simulink model "Ctrl_For_HRV_alpha_reversal_harness"  (R2024b)
settings: Solver=ode4  StartTime=0.0  StopTime=100  FixedStep=0.02  RelTol=1e-3
InitFcn:
  | Parameter;
values from neighbouring files (symbols this model uses):
  h_alpha = 0.02    [Data_0.mat]    (also in Parameter.m)
  h_beta = 0.02    [Data_0.mat]    (also in Parameter.m)
  h_miu = 0.02    [Data_0.mat]    (also in Parameter.m)
  h_p = 0.02    [Data_0.mat]    (also in Parameter.m)
  h_q = 0.02    [Data_0.mat]    (also in Parameter.m)
  h_r = 0.02    [Data_0.mat]    (also in Parameter.m)
  r_alpha = 0.04    [Data_0.mat]    (also in Parameter.m)
  r_beta = 0.04    [Data_0.mat]    (also in Parameter.m)
  r_miu = 0.03    [Data_0.mat]    (also in Parameter.m = 0.24)
  r_p = 1.28    [Data_0.mat]    (also in Parameter.m)
  r_q = 1.28    [Data_0.mat]    (also in Parameter.m)
  r_r = 1.28    [Data_0.mat]    (also in Parameter.m)
  xishu = 0.3    [Data_0.mat]    (also in Parameter.m = 0)
  xishu_D_0 = 0.3    [Parameter.m]
  xishu_L_0 = 0.2    [Parameter.m]
  xishu_l_0 = 0.23    [Parameter.m]
  xishu_m_0 = 0.17    [Parameter.m]
  xishu_n_0 = 0.09    [Parameter.m]
  xishu_Y_0 = 0.14    [Parameter.m]
undefined symbols (not defined in the file or in its folder): AngleRate_Controller, fhan, FlowAngle_Controller
libraries: simulink x12
settings Model: Creator=BinRen  LastModifiedBy=DuY
settings SolverCC: AlgebraicLoopSolver=TrustRegion
settings DataIOCC: SaveFormat=StructureWithTime  SaveState=on  TimeSaveName=time
settings DebuggingCC: UnconnectedInputMsg=warning  UnconnectedOutputMsg=warning  UnconnectedLineMsg=warning
settings ModelReferenceCC: EnableRefExpFcnMdlSchedulingChecks=on
settings RTWCC: GPUComputeCapability=3.5  DLArmComputeVersion=19.05

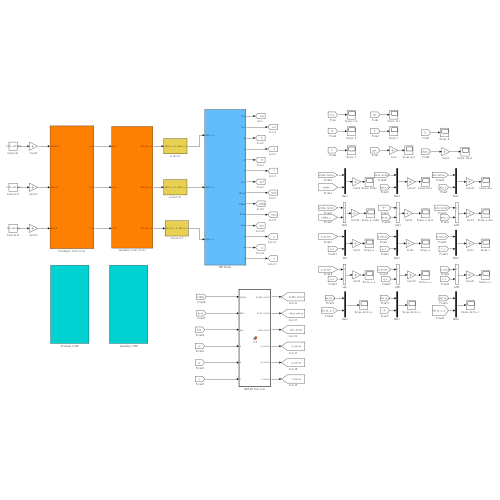
[thumbnail: Simulink's stored preview of the top-level diagram]
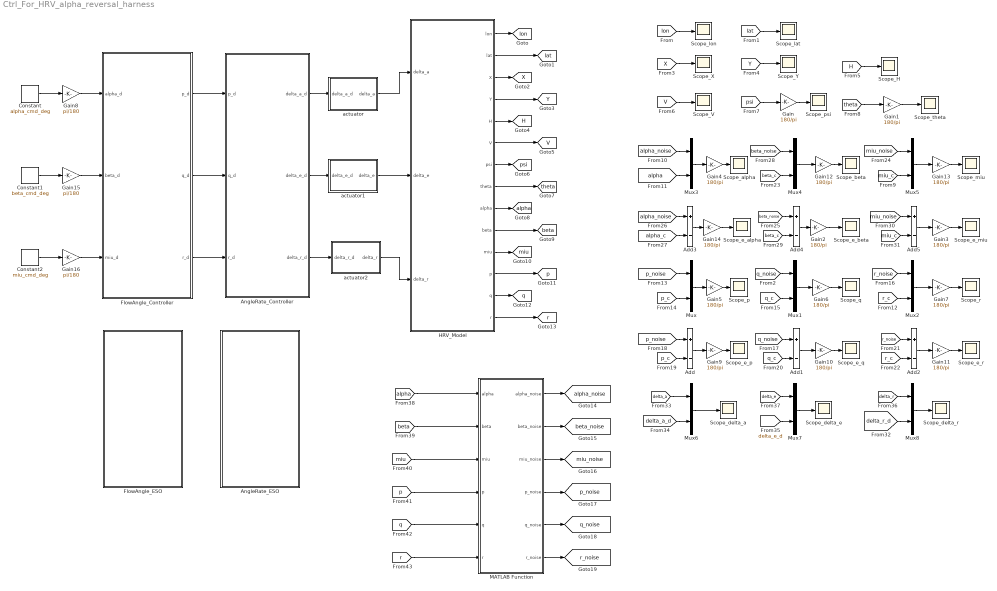
== system Ctrl_For_HRV_alpha_reversal_harness ==
  Add{,1..5} (6 alike) : Sum  Inputs=+-
  AngleRate_Controller : Subsystem
  AngleRate_ESO : Subsystem
  Constant : FromWorkspace  VariableName=alpha_cmd_deg
  Constant1 : FromWorkspace  VariableName=beta_cmd_deg
  Constant2 : FromWorkspace  VariableName=miu_cmd_deg
  FlowAngle_Controller : Subsystem
  FlowAngle_ESO : Subsystem
  Gain{,1..7,9..14} (14 alike) : Gain  Gain=180/pi
  Gain15 : Gain  Gain=pi/180
  Gain16 : Gain  Gain=pi/180
  Gain8 : Gain  Gain=pi/180
  HRV_Model : Subsystem
  MATLAB Function : MATLAB Function  TreatAsAtomicUnit=on
  Mux{,1..8} (9 alike) : Mux  Inputs=2
  Scope_H : Scope
  Scope_V : Scope
  Scope_X : Scope
  Scope_Y : Scope
  Scope_alpha : Scope
  Scope_beta : Scope
  Scope_delta_a : Scope
  Scope_delta_e : Scope
  Scope_delta_r : Scope
  Scope_e_alpha : Scope
  Scope_e_beta : Scope
  Scope_e_miu : Scope
  Scope_e_p : Scope
  Scope_e_q : Scope
  Scope_e_r : Scope
  Scope_lat : Scope
  Scope_lon : Scope
  Scope_miu : Scope
  Scope_p : Scope
  Scope_psi : Scope
  Scope_q : Scope
  Scope_r : Scope
  Scope_theta : Scope
  actuator : Subsystem
  actuator1 : Subsystem
  actuator2 : Subsystem
  tag scope: H=global, V=global, X=global, Y=global, alpha=global, alpha_noise=global, beta=global, beta_noise=global, lat=global, lon=global, miu=global, miu_noise=global, p=global, p_noise=global, psi=global, q=global, q_noise=global, r=global, r_noise=global, theta=global
  wires:
  HRV_Model/1(lon) -> [lon]
  HRV_Model/2(lat) -> [lat]
  HRV_Model/4(Y) -> [Y]
  HRV_Model/3(X) -> [X]
  HRV_Model/7(psi) -> [psi]
  HRV_Model/8(theta) -> [theta]
  HRV_Model/6(V) -> [V]
  HRV_Model/5(H) -> [H]
  HRV_Model/13(q) -> [q]
  HRV_Model/14(r) -> [r]
  HRV_Model/11(miu) -> [miu]
  HRV_Model/12(p) -> [p]
  HRV_Model/10(beta) -> [beta]
  HRV_Model/9(alpha) -> [alpha]
  [lon] -> Scope_lon/1
  [lat] -> Scope_lat/1
  [H] -> Scope_H/1
  [Y] -> Scope_Y/1
  [X] -> Scope_X/1
  [V] -> Scope_V/1
  [psi] -> Gain/1
  Gain/1 -> Scope_psi/1
  Gain1/1 -> Scope_theta/1
  [theta] -> Gain1/1
  Gain5/1 -> Scope_p/1
  Gain6/1 -> Scope_q/1
  Gain7/1 -> Scope_r/1
  actuator/1(delta_a) -> HRV_Model/1(delta_a)
  actuator1/1(delta_e) -> HRV_Model/2(delta_e)
  actuator2/1(delta_r) -> HRV_Model/3(delta_r)
  AngleRate_Controller/2(delta_e_d) -> actuator1/1(delta_e_d)
  [p_noise] -> Mux/1
  Mux/1 -> Gain5/1
  [p_c] -> Mux/2
  [q_c] -> Mux1/2
  [q_noise] -> Mux1/1
  Mux1/1 -> Gain6/1
  Mux2/1 -> Gain7/1
  [r_noise] -> Mux2/1
  [r_c] -> Mux2/2
  Gain11/1 -> Scope_e_r/1
  Gain10/1 -> Scope_e_q/1
  Gain9/1 -> Scope_e_p/1
  [p_c] -> Add/2
  [p_noise] -> Add/1
  Add/1 -> Gain9/1
  Add1/1 -> Gain10/1
  [q_noise] -> Add1/1
  [q_c] -> Add1/2
  [r_c] -> Add2/2
  [r_noise] -> Add2/1
  Add2/1 -> Gain11/1
  Add5/1 -> Gain3/1
  [miu_noise] -> Add5/1
  [miu_c] -> Add5/2
  [beta_c] -> Add4/2
  [beta_noise] -> Add4/1
  Add4/1 -> Gain2/1
  Add3/1 -> Gain14/1
  [alpha_noise] -> Add3/1
  [alpha_c] -> Add3/2
  Gain14/1 -> Scope_e_alpha/1
  Gain2/1 -> Scope_e_beta/1
  Gain3/1 -> Scope_e_miu/1
  [miu_c] -> Mux5/2
  [miu_noise] -> Mux5/1
  Mux5/1 -> Gain13/1
  Mux4/1 -> Gain12/1
  [beta_noise] -> Mux4/1
  [beta_c] -> Mux4/2
  [alpha] -> Mux3/2
  Mux3/1 -> Gain4/1
  [alpha_noise] -> Mux3/1
  Gain13/1 -> Scope_miu/1
  Gain12/1 -> Scope_beta/1
  Gain4/1 -> Scope_alpha/1
  Gain8/1 -> FlowAngle_Controller/1(alpha_d)
  [delta_r_d] -> Mux8/2
  [delta_r] -> Mux8/1
  [delta_e] -> Mux7/1
  [delta_e_d] -> Mux7/2
  [delta_a_d] -> Mux6/2
  [delta_a] -> Mux6/1
  Mux8/1 -> Scope_delta_r/1
  Mux7/1 -> Scope_delta_e/1
  Mux6/1 -> Scope_delta_a/1
  FlowAngle_Controller/1(p_d) -> AngleRate_Controller/1(p_d)
  FlowAngle_Controller/2(q_d) -> AngleRate_Controller/2(q_d)
  FlowAngle_Controller/3(r_d) -> AngleRate_Controller/3(r_d)
  Gain15/1 -> FlowAngle_Controller/2(beta_d)
  Gain16/1 -> FlowAngle_Controller/3(miu_d)
  AngleRate_Controller/3(delta_r_d) -> actuator2/1(delta_r_d)
  AngleRate_Controller/1(delta_a_d) -> actuator/1(delta_a_d)
  MATLAB Function/1(alpha_noise) -> [alpha_noise]
  [alpha] -> MATLAB Function/1(alpha)
  [beta] -> MATLAB Function/2(beta)
  [miu] -> MATLAB Function/3(miu)
  [p] -> MATLAB Function/4(p)
  [q] -> MATLAB Function/5(q)
  [r] -> MATLAB Function/6(r)
  MATLAB Function/2(beta_noise) -> [beta_noise]
  MATLAB Function/3(miu_noise) -> [miu_noise]
  MATLAB Function/4(p_noise) -> [p_noise]
  MATLAB Function/5(q_noise) -> [q_noise]
  MATLAB Function/6(r_noise) -> [r_noise]
  Constant/1 -> Gain8/1
  Constant1/1 -> Gain15/1
  Constant2/1 -> Gain16/1

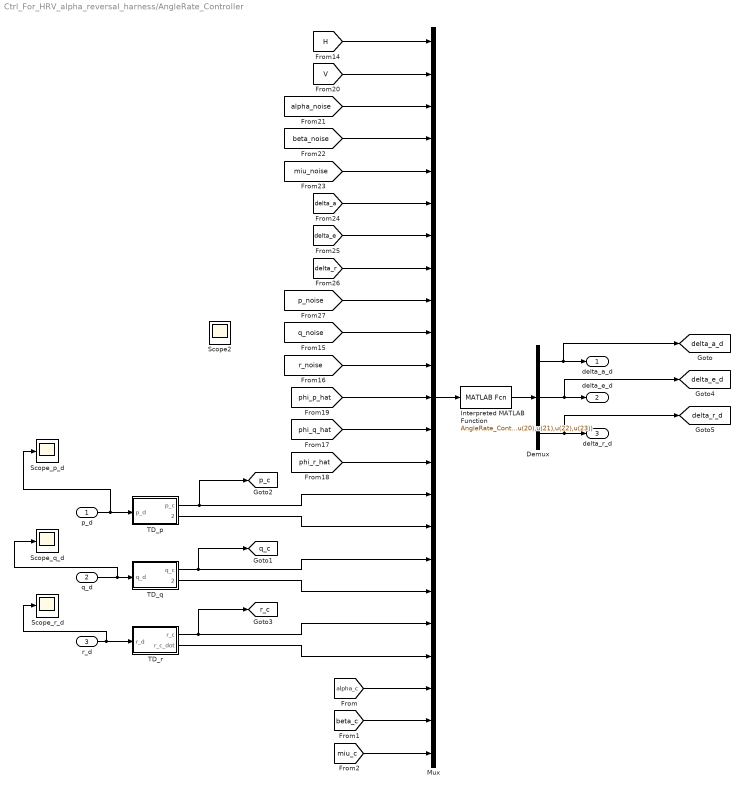
== system Ctrl_For_HRV_alpha_reversal_harness/AngleRate_Controller ==
  p_d : Inport
  q_d : Inport  Port=2
  r_d : Inport  Port=3
  Demux : Demux  Outputs=3
  Interpreted MATLAB Function : MATLABFcn  MATLABFcn=AngleRate_Controller(u(1),u(2),u(3),u(4),u(5),u(6),u(7),u(8),u(9),u(10),u(11),u(12),u(13),u(14),u(15),u(16),u(17),u(18),u(19),u(20),u(21),u(22),u(23))  OutputDimensions=3
  Mux : Mux  Inputs=23
  Scope2 : Scope
  Scope_p_d : Scope
  Scope_q_d : Scope
  Scope_r_d : Scope
  TD_p : Subsystem
  TD_q : Subsystem
  TD_r : Subsystem
  delta_a_d : Outport
  delta_e_d : Outport  Port=2
  delta_r_d : Outport  Port=3
  tag scope: delta_a_d=global, delta_e_d=global, delta_r_d=global, p_c=global, q_c=global, r_c=global
  wires:
  [miu_noise] -> Mux/5
  [beta_noise] -> Mux/4
  TD_r/1(r_c) -> [r_c], Mux/19
  TD_p/2(p_c_dot) -> Mux/16
  TD_q/2(q_c_dot) -> Mux/18
  [q_noise] -> Mux/10
  TD_q/1(q_c) -> [q_c], Mux/17
  TD_r/2(r_c_dot) -> Mux/20
  [r_noise] -> Mux/11
  [H] -> Mux/1
  [p_noise] -> Mux/9
  [V] -> Mux/2
  [alpha_noise] -> Mux/3
  Mux/1 -> Interpreted MATLAB Function/1
  Interpreted MATLAB Function/1 -> Demux/1
  [delta_a] -> Mux/6
  [delta_r] -> Mux/8
  [delta_e] -> Mux/7
  TD_p/1(p_c) -> [p_c], Mux/15
  Demux/3 -> [delta_r_d], delta_r_d/1
  r_d/1 -> Scope_r_d/1, TD_r/1(r_d)
  Demux/2 -> [delta_e_d], delta_e_d/1
  Demux/1 -> [delta_a_d], delta_a_d/1
  q_d/1 -> Scope_q_d/1, TD_q/1(q_d)
  p_d/1 -> Scope_p_d/1, TD_p/1(p_d)
  [phi_p_hat] -> Mux/12
  [phi_q_hat] -> Mux/13
  [phi_r_hat] -> Mux/14
  [alpha_c] -> Mux/21
  [beta_c] -> Mux/22
  [miu_c] -> Mux/23

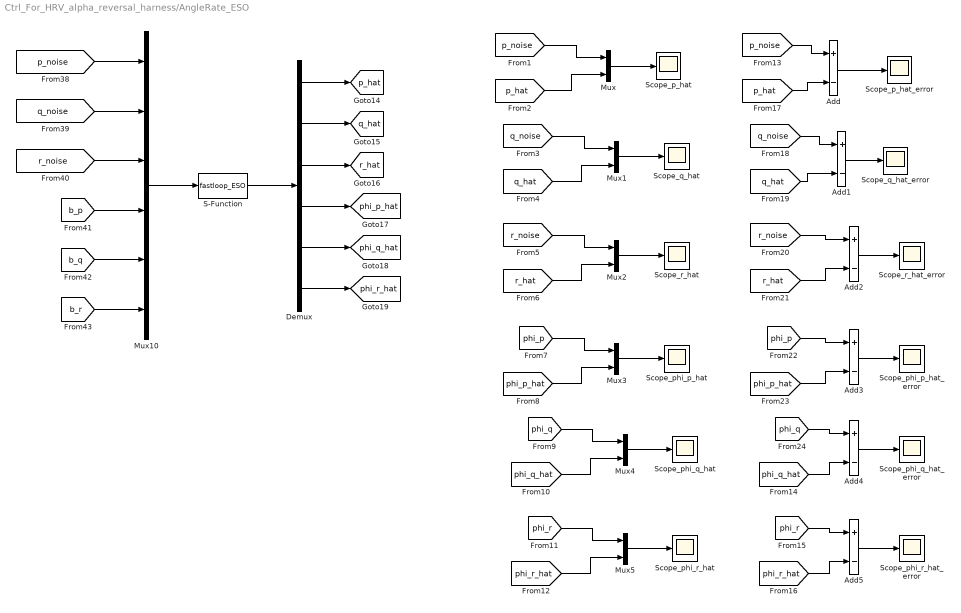
== system Ctrl_For_HRV_alpha_reversal_harness/AngleRate_ESO ==
  Add{,1..5} (6 alike) : Sum  Inputs=+-
  Demux : Demux  Outputs=6
  Mux{,1..5} (6 alike) : Mux  Inputs=2
  Mux10 : Mux  Inputs=6
  S-Function : S-Function  FunctionName=fastloop_ESO  SFunctionDeploymentMode=off  EnableBusSupport=off
  Scope_p_hat : Scope
  Scope_p_hat_error : Scope
  Scope_phi_p_hat : Scope
  Scope_phi_p_hat_error : Scope
  Scope_phi_q_hat : Scope
  Scope_phi_q_hat_error : Scope
  Scope_phi_r_hat : Scope
  Scope_phi_r_hat_error : Scope
  Scope_q_hat : Scope
  Scope_q_hat_error : Scope
  Scope_r_hat : Scope
  Scope_r_hat_error : Scope
  tag scope: p_hat=global, phi_p_hat=global, phi_q_hat=global, phi_r_hat=global, q_hat=global, r_hat=global
  wires:
  [b_q] -> Mux10/5
  [r_noise] -> Mux10/3
  [q_noise] -> Mux10/2
  Demux/2 -> [q_hat]
  [b_p] -> Mux10/4
  S-Function/1 -> Demux/1
  Demux/5 -> [phi_q_hat]
  Demux/1 -> [p_hat]
  Demux/3 -> [r_hat]
  Demux/4 -> [phi_p_hat]
  Mux10/1 -> S-Function/1
  Demux/6 -> [phi_r_hat]
  [p_noise] -> Mux10/1
  [b_r] -> Mux10/6
  Mux/1 -> Scope_p_hat/1
  [p_noise] -> Mux/1
  [p_hat] -> Mux/2
  [q_noise] -> Mux1/1
  [q_hat] -> Mux1/2
  Mux1/1 -> Scope_q_hat/1
  [r_noise] -> Mux2/1
  [r_hat] -> Mux2/2
  Mux2/1 -> Scope_r_hat/1
  Mux5/1 -> Scope_phi_r_hat/1
  [phi_r_hat] -> Mux5/2
  [phi_r] -> Mux5/1
  Mux4/1 -> Scope_phi_q_hat/1
  [phi_q_hat] -> Mux4/2
  [phi_q] -> Mux4/1
  [phi_p_hat] -> Mux3/2
  [phi_p] -> Mux3/1
  Mux3/1 -> Scope_phi_p_hat/1
  [p_noise] -> Add/1
  [p_hat] -> Add/2
  Add/1 -> Scope_p_hat_error/1
  [q_noise] -> Add1/1
  [q_hat] -> Add1/2
  Add1/1 -> Scope_q_hat_error/1
  [r_noise] -> Add2/1
  [r_hat] -> Add2/2
  Add2/1 -> Scope_r_hat_error/1
  [phi_p] -> Add3/1
  [phi_p_hat] -> Add3/2
  Add3/1 -> Scope_phi_p_hat_error/1
  [phi_q] -> Add4/1
  [phi_q_hat] -> Add4/2
  Add4/1 -> Scope_phi_q_hat_error/1
  [phi_r] -> Add5/1
  [phi_r_hat] -> Add5/2
  Add5/1 -> Scope_phi_r_hat_error/1

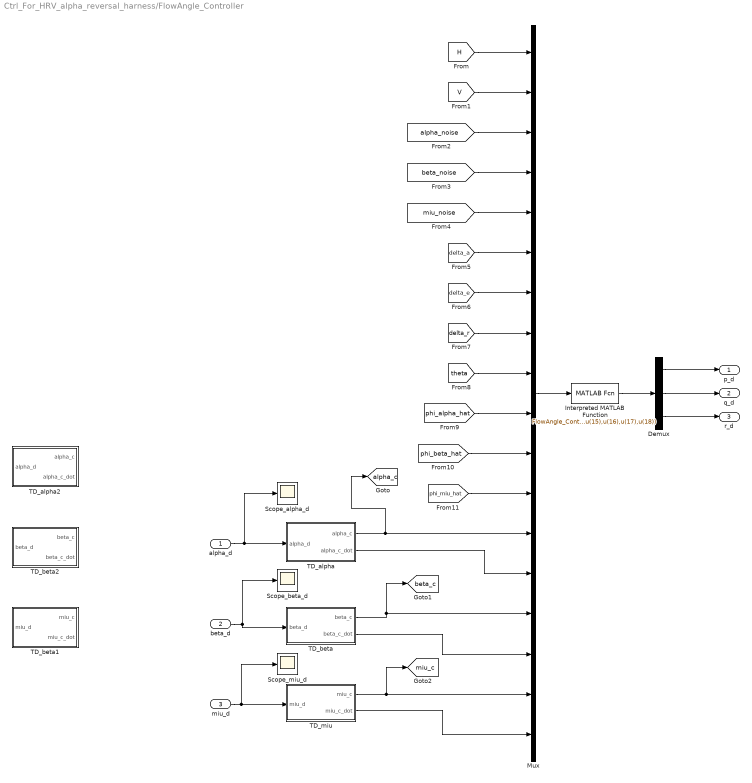
== system Ctrl_For_HRV_alpha_reversal_harness/FlowAngle_Controller ==
  alpha_d : Inport
  beta_d : Inport  Port=2
  miu_d : Inport  Port=3
  Demux : Demux  Outputs=3
  Interpreted MATLAB Function : MATLABFcn  MATLABFcn=FlowAngle_Controller(u(1),u(2),u(3),u(4),u(5),u(6),u(7),u(8),u(9),u(10),u(11),u(12),u(13),u(14),u(15),u(16),u(17),u(18))  OutputDimensions=3
  Mux : Mux  Inputs=18
  Scope_alpha_d : Scope
  Scope_beta_d : Scope
  Scope_miu_d : Scope
  TD_alpha : Subsystem
  TD_alpha2 : Subsystem
  TD_beta : Subsystem
  TD_beta1 : Subsystem
  TD_beta2 : Subsystem
  TD_miu : Subsystem
  p_d : Outport
  q_d : Outport  Port=2
  r_d : Outport  Port=3
  tag scope: alpha_c=global, beta_c=global, miu_c=global
  wires:
  [H] -> Mux/1
  [V] -> Mux/2
  [alpha_noise] -> Mux/3
  [beta_noise] -> Mux/4
  [miu_noise] -> Mux/5
  [delta_r] -> Mux/8
  [delta_e] -> Mux/7
  [delta_a] -> Mux/6
  [theta] -> Mux/9
  Mux/1 -> Interpreted MATLAB Function/1
  Interpreted MATLAB Function/1 -> Demux/1
  Demux/1 -> p_d/1
  Demux/2 -> q_d/1
  Demux/3 -> r_d/1
  alpha_d/1 -> Scope_alpha_d/1, TD_alpha/1(alpha_d)
  TD_alpha/1(alpha_c) -> [alpha_c], Mux/13
  TD_alpha/2(alpha_c_dot) -> Mux/14
  beta_d/1 -> Scope_beta_d/1, TD_beta/1(beta_d)
  TD_beta/1(beta_c) -> [beta_c], Mux/15
  TD_beta/2(beta_c_dot) -> Mux/16
  miu_d/1 -> Scope_miu_d/1, TD_miu/1(miu_d)
  TD_miu/1(miu_c) -> [miu_c], Mux/17
  TD_miu/2(miu_c_dot) -> Mux/18
  [phi_alpha_hat] -> Mux/10
  [phi_beta_hat] -> Mux/11
  [phi_miu_hat] -> Mux/12

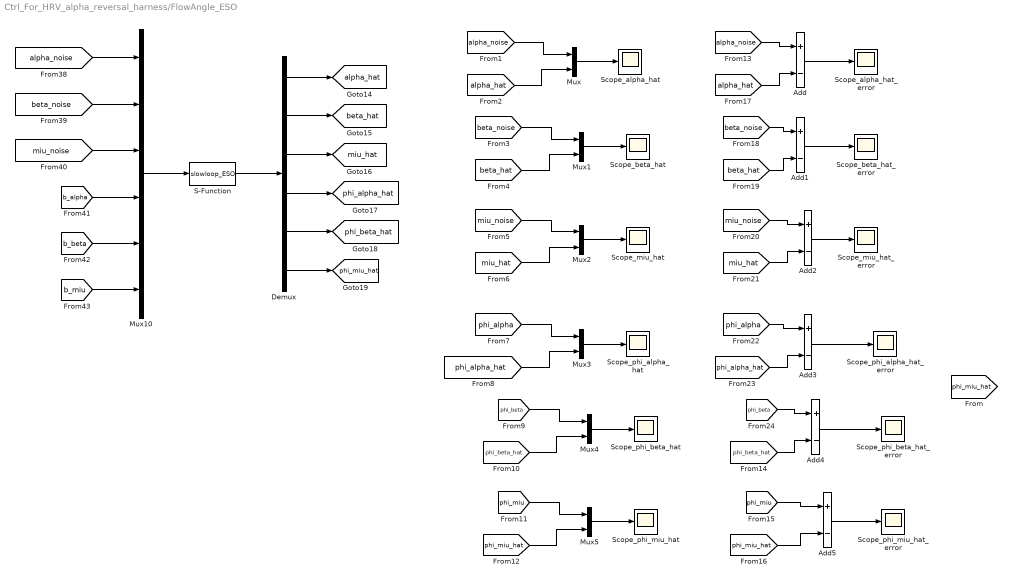
== system Ctrl_For_HRV_alpha_reversal_harness/FlowAngle_ESO ==
  Add{,1..5} (6 alike) : Sum  Inputs=+-
  Demux : Demux  Outputs=6
  Mux{,1..5} (6 alike) : Mux  Inputs=2
  Mux10 : Mux  Inputs=6
  S-Function : S-Function  FunctionName=slowloop_ESO  SFunctionDeploymentMode=off  EnableBusSupport=off
  Scope_alpha_hat : Scope
  Scope_alpha_hat_error : Scope
  Scope_beta_hat : Scope
  Scope_beta_hat_error : Scope
  Scope_miu_hat : Scope
  Scope_miu_hat_error : Scope
  Scope_phi_alpha_hat : Scope
  Scope_phi_alpha_hat_error : Scope
  Scope_phi_beta_hat : Scope
  Scope_phi_beta_hat_error : Scope
  Scope_phi_miu_hat : Scope
  Scope_phi_miu_hat_error : Scope
  tag scope: alpha_hat=global, beta_hat=global, miu_hat=global, phi_alpha_hat=global, phi_beta_hat=global, phi_miu_hat=global
  wires:
  [b_beta] -> Mux10/5
  [miu_noise] -> Mux10/3
  [beta_noise] -> Mux10/2
  Demux/2 -> [beta_hat]
  [b_alpha] -> Mux10/4
  S-Function/1 -> Demux/1
  Demux/5 -> [phi_beta_hat]
  Demux/1 -> [alpha_hat]
  Demux/3 -> [miu_hat]
  Demux/4 -> [phi_alpha_hat]
  Mux10/1 -> S-Function/1
  Demux/6 -> [phi_miu_hat]
  [alpha_noise] -> Mux10/1
  [b_miu] -> Mux10/6
  Mux/1 -> Scope_alpha_hat/1
  [alpha_noise] -> Mux/1
  [alpha_hat] -> Mux/2
  [beta_noise] -> Mux1/1
  [beta_hat] -> Mux1/2
  Mux1/1 -> Scope_beta_hat/1
  [miu_noise] -> Mux2/1
  [miu_hat] -> Mux2/2
  Mux2/1 -> Scope_miu_hat/1
  Mux5/1 -> Scope_phi_miu_hat/1
  [phi_miu_hat] -> Mux5/2
  [phi_miu] -> Mux5/1
  Mux4/1 -> Scope_phi_beta_hat/1
  [phi_beta_hat] -> Mux4/2
  [phi_beta] -> Mux4/1
  [phi_alpha_hat] -> Mux3/2
  [phi_alpha] -> Mux3/1
  Mux3/1 -> Scope_phi_alpha_hat/1
  [alpha_noise] -> Add/1
  [alpha_hat] -> Add/2
  Add/1 -> Scope_alpha_hat_error/1
  [beta_noise] -> Add1/1
  [beta_hat] -> Add1/2
  Add1/1 -> Scope_beta_hat_error/1
  [miu_noise] -> Add2/1
  [miu_hat] -> Add2/2
  Add2/1 -> Scope_miu_hat_error/1
  [phi_alpha] -> Add3/1
  [phi_alpha_hat] -> Add3/2
  Add3/1 -> Scope_phi_alpha_hat_error/1
  [phi_beta] -> Add4/1
  [phi_beta_hat] -> Add4/2
  Add4/1 -> Scope_phi_beta_hat_error/1
  Add5/1 -> Scope_phi_miu_hat_error/1
  [phi_miu] -> Add5/1
  [phi_miu_hat] -> Add5/2

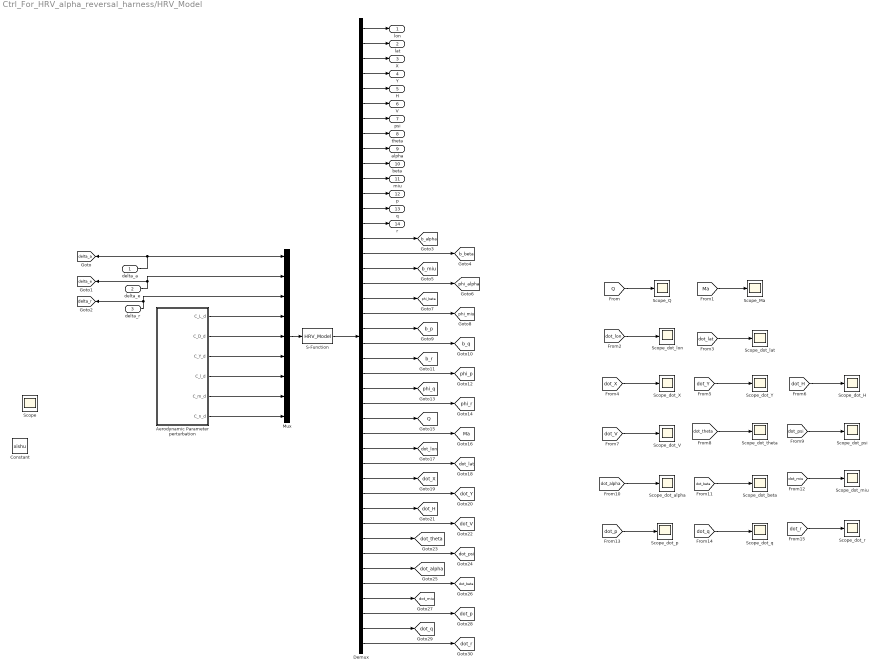
== system Ctrl_For_HRV_alpha_reversal_harness/HRV_Model ==
  delta_a : Inport
  delta_e : Inport  Port=2
  delta_r : Inport  Port=3
  Aerodynamic Parameter perturbation : Subsystem
  Constant : Constant  Value=xishu  SampleTime=-1
  Demux : Demux  Outputs=14 + 12 + 2 + 14
  Mux : Mux  Inputs=9
  S-Function : S-Function  FunctionName=HRV_Model  SFunctionDeploymentMode=off  EnableBusSupport=off
  Scope : Scope
  Scope_Ma : Scope
  Scope_Q : Scope
  Scope_dot_H : Scope
  Scope_dot_V : Scope
  Scope_dot_X : Scope
  Scope_dot_Y : Scope
  Scope_dot_alpha : Scope
  Scope_dot_beta : Scope
  Scope_dot_lat : Scope
  Scope_dot_lon : Scope
  Scope_dot_miu : Scope
  Scope_dot_p : Scope
  Scope_dot_psi : Scope
  Scope_dot_q : Scope
  Scope_dot_r : Scope
  Scope_dot_theta : Scope
  lon : Outport
  lat : Outport  Port=2
  X : Outport  Port=3
  Y : Outport  Port=4
  H : Outport  Port=5
  V : Outport  Port=6
  psi : Outport  Port=7
  theta : Outport  Port=8
  alpha : Outport  Port=9
  beta : Outport  Port=10
  miu : Outport  Port=11
  p : Outport  Port=12
  q : Outport  Port=13
  r : Outport  Port=14
  tag scope: Ma=global, Q=global, b_alpha=global, b_beta=global, b_miu=global, b_p=global, b_q=global, b_r=global, delta_a=global, delta_e=global, delta_r=global, dot_H=global, dot_V=global, dot_X=global, dot_Y=global, dot_alpha=global, dot_beta=global, dot_lat=global, dot_lon=global, dot_miu=global, dot_p=global, dot_psi=global, dot_q=global, dot_r=global, dot_theta=global, phi_alpha=global, phi_beta=global, phi_miu=global, phi_p=global, phi_q=global, phi_r=global
  wires:
  Demux/8 -> theta/1
  Mux/1 -> S-Function/1
  S-Function/1 -> Demux/1
  Demux/1 -> lon/1
  Demux/2 -> lat/1
  Demux/3 -> X/1
  Demux/7 -> psi/1
  Demux/11 -> miu/1
  Demux/10 -> beta/1
  Demux/9 -> alpha/1
  Demux/12 -> p/1
  Demux/5 -> H/1
  delta_e/1 -> [delta_e], Mux/2
  Demux/6 -> V/1
  Demux/14 -> r/1
  delta_r/1 -> [delta_r], Mux/3
  Demux/13 -> q/1
  delta_a/1 -> [delta_a], Mux/1
  Demux/4 -> Y/1
  Demux/15 -> [b_alpha]
  Demux/16 -> [b_beta]
  Demux/18 -> [phi_alpha]
  Demux/17 -> [b_miu]
  Demux/21 -> [b_p]
  Demux/22 -> [b_q]
  Demux/20 -> [phi_miu]
  Demux/19 -> [phi_beta]
  Demux/23 -> [b_r]
  Demux/24 -> [phi_p]
  Demux/25 -> [phi_q]
  Demux/26 -> [phi_r]
  Demux/27 -> [Q]
  Demux/28 -> [Ma]
  Demux/30 -> [dot_lat]
  Demux/29 -> [dot_lon]
  Demux/31 -> [dot_X]
  Demux/32 -> [dot_Y]
  Demux/37 -> [dot_alpha]
  Demux/36 -> [dot_psi]
  Demux/34 -> [dot_V]
  Demux/35 -> [dot_theta]
  Demux/33 -> [dot_H]
  Demux/39 -> [dot_miu]
  Demux/38 -> [dot_beta]
  Demux/40 -> [dot_p]
  Demux/41 -> [dot_q]
  Demux/42 -> [dot_r]
  [Q] -> Scope_Q/1
  [Ma] -> Scope_Ma/1
  [dot_lon] -> Scope_dot_lon/1
  [dot_lat] -> Scope_dot_lat/1
  [dot_X] -> Scope_dot_X/1
  [dot_Y] -> Scope_dot_Y/1
  [dot_H] -> Scope_dot_H/1
  [dot_V] -> Scope_dot_V/1
  [dot_theta] -> Scope_dot_theta/1
  [dot_psi] -> Scope_dot_psi/1
  [dot_alpha] -> Scope_dot_alpha/1
  [dot_beta] -> Scope_dot_beta/1
  [dot_miu] -> Scope_dot_miu/1
  [dot_r] -> Scope_dot_r/1
  [dot_q] -> Scope_dot_q/1
  [dot_p] -> Scope_dot_p/1
  Aerodynamic Parameter perturbation/1(C_L_d) -> Mux/4
  Aerodynamic Parameter perturbation/2(C_D_d) -> Mux/5
  Aerodynamic Parameter perturbation/3(C_Y_d) -> Mux/6
  Aerodynamic Parameter perturbation/4(C_l_d) -> Mux/7
  Aerodynamic Parameter perturbation/5(C_m_d) -> Mux/8
  Aerodynamic Parameter perturbation/6(C_n_d) -> Mux/9

== system Ctrl_For_HRV_alpha_reversal_harness/actuator ==
  delta_a_d : Inport
  Gain : Gain  Gain=50
  Integrator : Integrator
  Saturation : Saturate  UpperLimit=90  LowerLimit=-90
  Saturation1 : Saturate  UpperLimit=30  LowerLimit=-30
  Sum : Sum  Inputs=|+-
  delta_a : Outport
  wires:
  Saturation/1 -> Integrator/1
  Sum/1 -> Gain/1
  Integrator/1 -> Saturation1/1, Sum/2
  delta_a_d/1 -> Sum/1
  Gain/1 -> Saturation/1
  Saturation1/1 -> delta_a/1

== system Ctrl_For_HRV_alpha_reversal_harness/actuator1 ==
  delta_e_d : Inport
  Gain : Gain  Gain=50
  Integrator : Integrator
  Saturation : Saturate  UpperLimit=90  LowerLimit=-90
  Saturation1 : Saturate  UpperLimit=30  LowerLimit=-30
  Sum : Sum  Inputs=|+-
  delta_e : Outport
  wires:
  Saturation1/1 -> delta_e/1
  Gain/1 -> Saturation/1
  delta_e_d/1 -> Sum/1
  Integrator/1 -> Sum/2, Saturation1/1
  Sum/1 -> Gain/1
  Saturation/1 -> Integrator/1

== system Ctrl_For_HRV_alpha_reversal_harness/actuator2 ==
  delta_r_d : Inport
  Gain : Gain  Gain=50
  Integrator : Integrator
  Saturation : Saturate  UpperLimit=90  LowerLimit=-90
  Saturation1 : Saturate  UpperLimit=30  LowerLimit=-30
  Sum : Sum  Inputs=|+-
  delta_r : Outport
  wires:
  Saturation/1 -> Integrator/1
  Sum/1 -> Gain/1
  Integrator/1 -> Saturation1/1, Sum/2
  delta_r_d/1 -> Sum/1
  Gain/1 -> Saturation/1
  Saturation1/1 -> delta_r/1

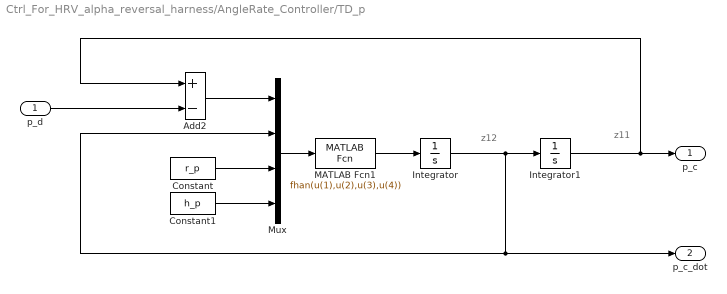
== system Ctrl_For_HRV_alpha_reversal_harness/AngleRate_Controller/TD_p ==
  note: z11
  note: z12
  p_d : Inport
  Add2 : Sum  Inputs=+-
  Constant : Constant  Value=r_p
  Constant1 : Constant  Value=h_p
  Integrator : Integrator
  Integrator1 : Integrator
  MATLAB Fcn1 : MATLABFcn  MATLABFcn=fhan(u(1),u(2),u(3),u(4))
  Mux : Mux
  p_c : Outport  VectorParamsAs1DForOutWhenUnconnected=off
  p_c_dot : Outport  Port=2  VectorParamsAs1DForOutWhenUnconnected=off
  wires:
  Integrator/1 -> Integrator1/1, p_c_dot/1, Mux/2
  Integrator1/1 -> Add2/1, p_c/1
  MATLAB Fcn1/1 -> Integrator/1
  Mux/1 -> MATLAB Fcn1/1
  Constant/1 -> Mux/3
  Constant1/1 -> Mux/4
  Add2/1 -> Mux/1
  p_d/1 -> Add2/2

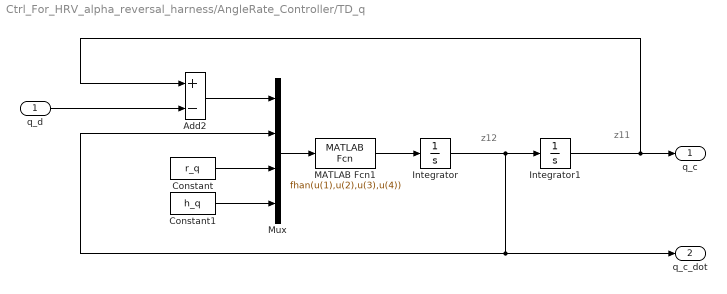
== system Ctrl_For_HRV_alpha_reversal_harness/AngleRate_Controller/TD_q ==
  note: z11
  note: z12
  q_d : Inport
  Add2 : Sum  Inputs=+-
  Constant : Constant  Value=r_q
  Constant1 : Constant  Value=h_q
  Integrator : Integrator
  Integrator1 : Integrator
  MATLAB Fcn1 : MATLABFcn  MATLABFcn=fhan(u(1),u(2),u(3),u(4))
  Mux : Mux
  q_c : Outport  VectorParamsAs1DForOutWhenUnconnected=off
  q_c_dot : Outport  Port=2  VectorParamsAs1DForOutWhenUnconnected=off
  wires:
  Integrator/1 -> Integrator1/1, q_c_dot/1, Mux/2
  Integrator1/1 -> Add2/1, q_c/1
  MATLAB Fcn1/1 -> Integrator/1
  Mux/1 -> MATLAB Fcn1/1
  Constant/1 -> Mux/3
  Constant1/1 -> Mux/4
  Add2/1 -> Mux/1
  q_d/1 -> Add2/2

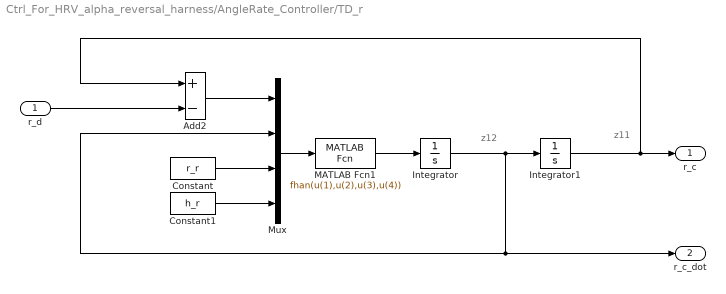
== system Ctrl_For_HRV_alpha_reversal_harness/AngleRate_Controller/TD_r ==
  note: z11
  note: z12
  r_d : Inport
  Add2 : Sum  Inputs=+-
  Constant : Constant  Value=r_r
  Constant1 : Constant  Value=h_r
  Integrator : Integrator
  Integrator1 : Integrator
  MATLAB Fcn1 : MATLABFcn  MATLABFcn=fhan(u(1),u(2),u(3),u(4))
  Mux : Mux
  r_c : Outport  VectorParamsAs1DForOutWhenUnconnected=off
  r_c_dot : Outport  Port=2  VectorParamsAs1DForOutWhenUnconnected=off
  wires:
  Integrator/1 -> Integrator1/1, r_c_dot/1, Mux/2
  Integrator1/1 -> Add2/1, r_c/1
  MATLAB Fcn1/1 -> Integrator/1
  Mux/1 -> MATLAB Fcn1/1
  Constant/1 -> Mux/3
  Constant1/1 -> Mux/4
  Add2/1 -> Mux/1
  r_d/1 -> Add2/2

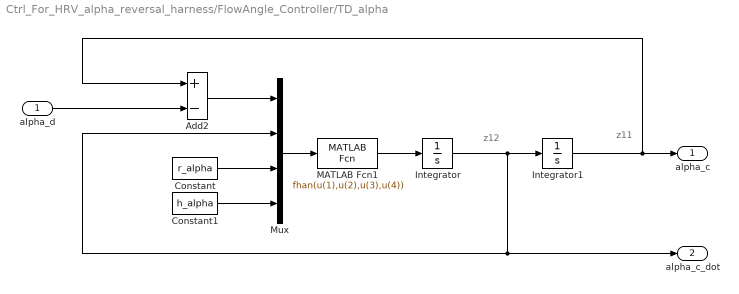
== system Ctrl_For_HRV_alpha_reversal_harness/FlowAngle_Controller/TD_alpha ==
  note: z11
  note: z12
  alpha_d : Inport
  Add2 : Sum  Inputs=+-
  Constant : Constant  Value=r_alpha
  Constant1 : Constant  Value=h_alpha
  Integrator : Integrator
  Integrator1 : Integrator
  MATLAB Fcn1 : MATLABFcn  MATLABFcn=fhan(u(1),u(2),u(3),u(4))
  Mux : Mux
  alpha_c : Outport  VectorParamsAs1DForOutWhenUnconnected=off
  alpha_c_dot : Outport  Port=2  VectorParamsAs1DForOutWhenUnconnected=off
  wires:
  Integrator/1 -> Integrator1/1, alpha_c_dot/1, Mux/2
  Integrator1/1 -> Add2/1, alpha_c/1
  MATLAB Fcn1/1 -> Integrator/1
  Mux/1 -> MATLAB Fcn1/1
  Constant/1 -> Mux/3
  Constant1/1 -> Mux/4
  Add2/1 -> Mux/1
  alpha_d/1 -> Add2/2

== system Ctrl_For_HRV_alpha_reversal_harness/FlowAngle_Controller/TD_alpha2 ==
  alpha_d : Inport
  Gain17 : Gain  Gain=1.2
  Integrator : Integrator
  Sum : Sum  Inputs=|+-
  alpha_c : Outport
  alpha_c_dot : Outport  Port=2
  wires:
  Gain17/1 -> alpha_c_dot/1, Integrator/1
  Integrator/1 -> alpha_c/1, Sum/2
  Sum/1 -> Gain17/1
  alpha_d/1 -> Sum/1

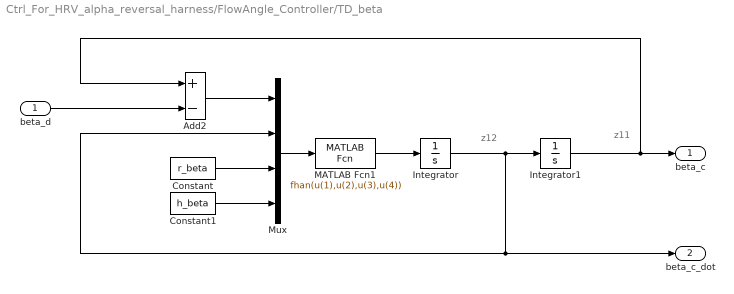
== system Ctrl_For_HRV_alpha_reversal_harness/FlowAngle_Controller/TD_beta ==
  note: z11
  note: z12
  beta_d : Inport
  Add2 : Sum  Inputs=+-
  Constant : Constant  Value=r_beta
  Constant1 : Constant  Value=h_beta
  Integrator : Integrator
  Integrator1 : Integrator
  MATLAB Fcn1 : MATLABFcn  MATLABFcn=fhan(u(1),u(2),u(3),u(4))
  Mux : Mux
  beta_c : Outport  VectorParamsAs1DForOutWhenUnconnected=off
  beta_c_dot : Outport  Port=2  VectorParamsAs1DForOutWhenUnconnected=off
  wires:
  Integrator/1 -> Integrator1/1, beta_c_dot/1, Mux/2
  Integrator1/1 -> Add2/1, beta_c/1
  MATLAB Fcn1/1 -> Integrator/1
  Mux/1 -> MATLAB Fcn1/1
  Constant/1 -> Mux/3
  Constant1/1 -> Mux/4
  Add2/1 -> Mux/1
  beta_d/1 -> Add2/2

== system Ctrl_For_HRV_alpha_reversal_harness/FlowAngle_Controller/TD_beta1 ==
  miu_d : Inport
  Gain17 : Gain  Gain=0.8
  Integrator : Integrator
  Sum : Sum  Inputs=|+-
  miu_c : Outport
  miu_c_dot : Outport  Port=2
  wires:
  Gain17/1 -> miu_c_dot/1, Integrator/1
  Integrator/1 -> miu_c/1, Sum/2
  Sum/1 -> Gain17/1
  miu_d/1 -> Sum/1

== system Ctrl_For_HRV_alpha_reversal_harness/FlowAngle_Controller/TD_beta2 ==
  beta_d : Inport
  Gain17 : Gain  Gain=1.2
  Integrator : Integrator
  Sum : Sum  Inputs=|+-
  beta_c : Outport
  beta_c_dot : Outport  Port=2
  wires:
  beta_d/1 -> Sum/1
  Sum/1 -> Gain17/1
  Integrator/1 -> Sum/2, beta_c/1
  Gain17/1 -> Integrator/1, beta_c_dot/1

== system Ctrl_For_HRV_alpha_reversal_harness/FlowAngle_Controller/TD_miu ==
  note: z11
  note: z12
  miu_d : Inport
  Add2 : Sum  Inputs=+-
  Constant : Constant  Value=r_miu
  Constant1 : Constant  Value=h_miu
  Integrator : Integrator
  Integrator1 : Integrator
  MATLAB Fcn1 : MATLABFcn  MATLABFcn=fhan(u(1),u(2),u(3),u(4))
  Mux : Mux
  miu_c : Outport  VectorParamsAs1DForOutWhenUnconnected=off
  miu_c_dot : Outport  Port=2  VectorParamsAs1DForOutWhenUnconnected=off
  wires:
  Integrator/1 -> Integrator1/1, miu_c_dot/1, Mux/2
  Integrator1/1 -> Add2/1, miu_c/1
  MATLAB Fcn1/1 -> Integrator/1
  Mux/1 -> MATLAB Fcn1/1
  Constant/1 -> Mux/3
  Constant1/1 -> Mux/4
  Add2/1 -> Mux/1
  miu_d/1 -> Add2/2

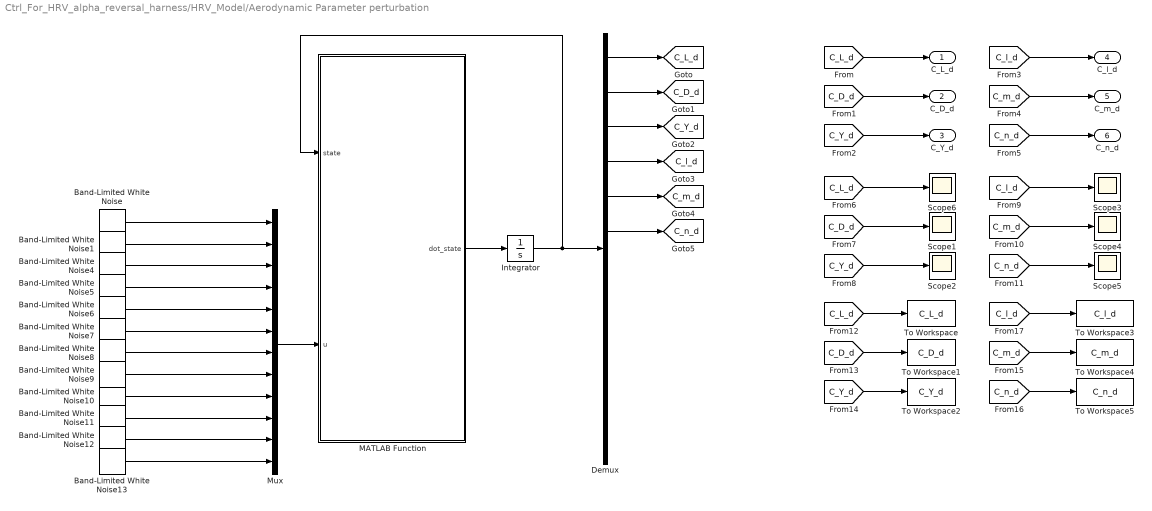
== system Ctrl_For_HRV_alpha_reversal_harness/HRV_Model/Aerodynamic Parameter perturbation ==
  Band-Limited White Noise{,1,4..7} (6 alike) : simulink/Sources/Band-Limited White Noise  Cov=1e-6  Ts=2  seed=round(rand()*1e5)
  Band-Limited White Noise{8..13} (6 alike) : simulink/Sources/Band-Limited White Noise  Cov=1e-10  Ts=2  seed=round(rand()*1e5)
  Demux : Demux  Outputs=12
  Integrator : Integrator  InitialCondition=[xishu_L_0,xishu_D_0,xishu_Y_0,xishu_l_0,xishu_m_0,xishu_n_0,0,0,0,0,0,0]
  MATLAB Function : MATLAB Function  TreatAsAtomicUnit=on
  Mux : Mux  Inputs=12
  Scope{1..6} (6 alike) : Scope
  To Workspace : ToWorkspace  VariableName=C_L_d  SampleTime=-1
      settings: Save2DSignal=2-D array (concatenate along first dimension)
  To Workspace1 : ToWorkspace  VariableName=C_D_d  SampleTime=-1
      settings: Save2DSignal=2-D array (concatenate along first dimension)
  To Workspace2 : ToWorkspace  VariableName=C_Y_d  SampleTime=-1
      settings: Save2DSignal=2-D array (concatenate along first dimension)
  To Workspace3 : ToWorkspace  VariableName=C_l_d  SampleTime=-1
      settings: Save2DSignal=2-D array (concatenate along first dimension)
  To Workspace4 : ToWorkspace  VariableName=C_m_d  SampleTime=-1
      settings: Save2DSignal=2-D array (concatenate along first dimension)
  To Workspace5 : ToWorkspace  VariableName=C_n_d  SampleTime=-1
      settings: Save2DSignal=2-D array (concatenate along first dimension)
  C_L_d : Outport
  C_D_d : Outport  Port=2
  C_Y_d : Outport  Port=3
  C_l_d : Outport  Port=4
  C_m_d : Outport  Port=5
  C_n_d : Outport  Port=6
  tag scope: C_D_d=global, C_L_d=global, C_Y_d=global, C_l_d=global, C_m_d=global, C_n_d=global
  wires:
  Mux/1 -> MATLAB Function/2(u)
  Band-Limited White Noise/1 -> Mux/1
  Band-Limited White Noise1/1 -> Mux/2
  Band-Limited White Noise5/1 -> Mux/4
  Band-Limited White Noise4/1 -> Mux/3
  Band-Limited White Noise6/1 -> Mux/5
  Band-Limited White Noise7/1 -> Mux/6
  Band-Limited White Noise8/1 -> Mux/7
  Band-Limited White Noise9/1 -> Mux/8
  Band-Limited White Noise10/1 -> Mux/9
  Band-Limited White Noise11/1 -> Mux/10
  Band-Limited White Noise12/1 -> Mux/11
  Band-Limited White Noise13/1 -> Mux/12
  MATLAB Function/1(dot_state) -> Integrator/1
  Integrator/1 -> Demux/1, MATLAB Function/1(state)
  Demux/1 -> [C_L_d]
  Demux/2 -> [C_D_d]
  Demux/3 -> [C_Y_d]
  Demux/4 -> [C_l_d]
  Demux/5 -> [C_m_d]
  Demux/6 -> [C_n_d]
  [C_L_d] -> C_L_d/1
  [C_D_d] -> C_D_d/1
  [C_Y_d] -> C_Y_d/1
  [C_l_d] -> C_l_d/1
  [C_m_d] -> C_m_d/1
  [C_n_d] -> C_n_d/1
  [C_Y_d] -> Scope2/1
  [C_m_d] -> Scope4/1
  [C_n_d] -> Scope5/1
  [C_l_d] -> Scope3/1
  [C_L_d] -> Scope6/1
  [C_D_d] -> Scope1/1
  [C_D_d] -> To Workspace1/1
  [C_L_d] -> To Workspace/1
  [C_Y_d] -> To Workspace2/1
  [C_l_d] -> To Workspace3/1
  [C_m_d] -> To Workspace4/1
  [C_n_d] -> To Workspace5/1

== matlab function Ctrl_For_HRV_alpha_reversal_harness/MATLAB Function ==
  settings: updateMethod=DISCRETE
  data: alpha input; alpha_noise output; beta input; miu input; p input; q input; r input; beta_noise output; miu_noise output; p_noise output; q_noise output; r_noise output
function [alpha_noise,beta_noise,miu_noise,p_noise,q_noise,r_noise]= fcn(alpha,beta,miu,p,q,r)

alpha_noise = awgn(alpha,80);
beta_noise = awgn(beta,100);
miu_noise = awgn(miu,100);
p_noise = awgn(p,100);
q_noise = awgn(q,100);
r_noise = awgn(r,100);

== matlab function Ctrl_For_HRV_alpha_reversal_harness/HRV_Model/Aerodynamic Parameter perturbation/MATLAB Function ==
  data: state input; dot_state output; u input
function dot_state  = Shedong_Model(state,u)
    C_L_d = state(1);C_D_d = state(2);C_Y_d = state(3);C_l_d = state(4);C_m_d = state(5);C_n_d = state(6);
    xi_L = state(7);xi_D = state(8);xi_Y = state(9);xi_l = state(10);xi_m = state(11);xi_n = state(12);
    omega_C_L_d = u(1);omega_C_D_d = u(2);omega_C_Y_d = u(3);omega_C_l_d = u(4);omega_C_m_d = u(5);omega_C_n_d = u(6);
    omega_xi_L_d = u(7);omega_xi_D_d = u(8);omega_xi_Y_d = u(9);omega_xi_l_d = u(10);omega_xi_m_d = u(11);omega_xi_n_d = u(12);

    dot_C_L_d = -xi_L*C_L_d+omega_C_L_d;    
    dot_C_D_d = -xi_D*C_D_d+omega_C_D_d;
    dot_C_Y_d = -xi_Y*C_Y_d+omega_C_Y_d;
    dot_C_l_d = -xi_l*C_l_d+omega_C_l_d;
    dot_C_m_d = -xi_m*C_m_d+omega_C_m_d;
    dot_C_n_d = -xi_n*C_n_d+omega_C_n_d;
    dot_xi_L = omega_xi_L_d;
    dot_xi_D = omega_xi_D_d;
    dot_xi_Y = omega_xi_Y_d;
    dot_xi_l = omega_xi_l_d;
    dot_xi_m = omega_xi_m_d;
    dot_xi_n = omega_xi_n_d;
            
    dot_state = [dot_C_L_d,dot_C_D_d,dot_C_Y_d,dot_C_l_d,dot_C_m_d,dot_C_n_d,dot_xi_L,dot_xi_D,dot_xi_Y,dot_xi_l,dot_xi_m,dot_xi_n];
end
